simulink model "noise"  (R2017b)
settings: Solver=FixedStepAuto  StartTime=0.0  StopTime=1000  FixedStep=0.01  MaxStep=0.01  RelTol=1e-3
settings Model: Creator=rablanco.ext  LastModifiedBy=rablanco.ext

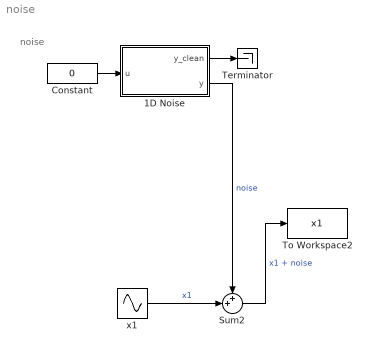
== system noise ==
  note: noise
  1D Noise : MATLAB Function  TreatAsAtomicUnit=on
  Constant : Constant  Value=0
  Sum2 : Sum  Inputs=++|
  Terminator : Terminator
  To Workspace2 : ToWorkspace  VariableName=x1  SampleTime=-1
  x1 : Sin  SampleTime=0
  wires:
  1D Noise/1(y_clean) -> Terminator/1
  Constant/1 -> 1D Noise/1(u)
  1D Noise/2(y) -> Sum2/1  "noise"
  x1/1 -> Sum2/2  "x1"
  Sum2/1 -> To Workspace2/1  "x1 + noise"

== matlab function noise/1D Noise ==
  data: y_clean output; u input; y output
function [y_clean,y] = fcn(u)
y_clean = u;
max_u=1;
noise = max_u.*.5.*(-1+2.*rand(1)); % rand num (-1,1)*(25% of u)->(-25%,25%) of u
y = u+ noise;
